simulink model "Ef_c"  (R2017a)
settings: Solver=VariableStepAuto  StartTime=0.0  StopTime=100  RelTol=1e-3
InitFcn:
  | m1 = .35;
  | m2 = 2;
  | l = .5;
  | g = 9.8;
  | ze = l/2;
  | 
  | C1 = 3/(m2*l^2+3*m1*ze^2);
  | 
  | tr_th = 1;
  | h_th = .707;
  | Wn_th = 2.2 / tr_th;
  | kd_th = 2*h_th*Wn_th/C1/l;
  | kp_th = Wn_th^2/(C1*l);
  | 
  | tr_z = 5*tr_th;
  | h = .707;
  | Wn = 2.2 / tr_z;
  | 
  | K = -Wn^2/9.81;
  | a = -K / ((1*h*Wn*1.5+.1)/(1.5*9.81));
  | K = -.022;
  | a = .3;
  | 
  | E_param
undefined symbols (not defined in the file or in its folder): E_animation, P
settings Model: Creator=Mat Haskell  LastModifiedBy=Mat Haskell

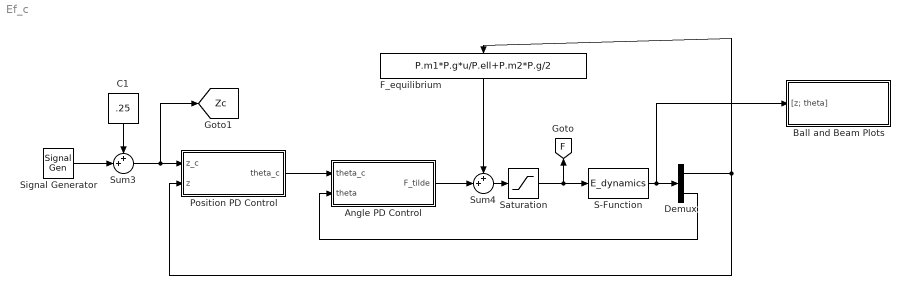
== system Ef_c ==
  Angle PD Control : Subsystem
  Ball and Beam Plots : Subsystem
  C1 : Constant  Value=.25
  Demux : Demux  Outputs=2
  F_equilibrium : Fcn  Expr=P.m1*P.g*u/P.ell+P.m2*P.g/2
  Position PD Control : Subsystem
  S-Function : S-Function  FunctionName=E_dynamics  Parameters=P  SFunctionDeploymentMode=off  EnableBusSupport=off
  Saturation : Saturate  UpperLimit=15  LowerLimit=0
  Signal Generator : SignalGenerator  WaveForm=square  Amplitude=.125  Frequency=.03
  Sum3 : Sum  Inputs=++|
  Sum4 : Sum  Inputs=++|
  tag scope: F=global, Zc=global
  wires:
  Sum4/1 -> Saturation/1
  F_equilibrium/1 -> Sum4/1
  Demux/2 -> Angle PD Control/2(theta)
  Position PD Control/1(theta_c) -> Angle PD Control/1(theta_c)
  Demux/1 -> Position PD Control/2(z), F_equilibrium/1
  Signal Generator/1 -> Sum3/2
  Sum3/1 -> [Zc], Position PD Control/1(z_c)
  Saturation/1 -> S-Function/1, [F]
  Angle PD Control/1(F_tilde) -> Sum4/2
  S-Function/1 -> Demux/1, Ball and Beam Plots/1("[z; theta]")
  C1/1 -> Sum3/1

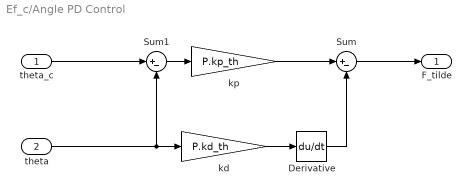
== system Ef_c/Angle PD Control ==
  theta_c : Inport
  theta : Inport  Port=2
  Derivative : Derivative
  Sum : Sum  Inputs=|+-
  Sum1 : Sum  Inputs=|+-
  kd : Gain  Gain=P.kd_th
  kp : Gain  Gain=P.kp_th
  F_tilde : Outport
  wires:
  Derivative/1 -> Sum/2
  Sum1/1 -> kp/1
  theta_c/1 -> Sum1/1
  Sum/1 -> F_tilde/1
  kp/1 -> Sum/1
  kd/1 -> Derivative/1
  theta/1 -> Sum1/2, kd/1

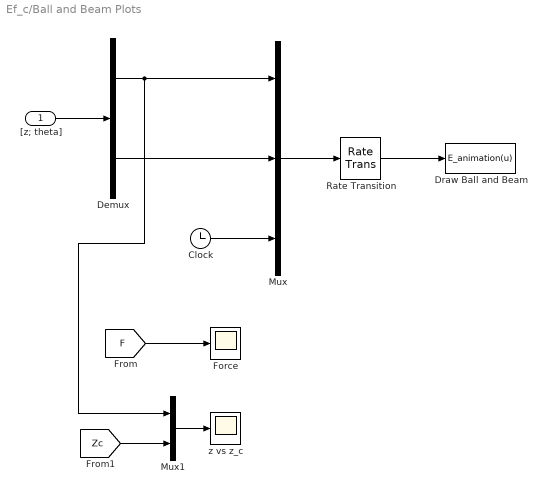
== system Ef_c/Ball and Beam Plots ==
  "[z; theta]" : Inport
  Clock : Clock
  Demux : Demux  Outputs=2
  Draw Ball and Beam : MATLABFcn  MATLABFcn=E_animation(u)  OutputDimensions=0
  Force : Scope
  Mux : Mux  Inputs=3
  Mux1 : Mux  Inputs=2
  Rate Transition : RateTransition  OutPortSampleTime=P.t_plot
  z vs z_c : Scope
  wires:
  "[z; theta]"/1 -> Demux/1
  Rate Transition/1 -> Draw Ball and Beam/1
  Mux/1 -> Rate Transition/1
  Clock/1 -> Mux/3
  Demux/1 -> Mux1/1, Mux/1
  Demux/2 -> Mux/2
  [F] -> Force/1
  Mux1/1 -> z vs z_c/1
  [Zc] -> Mux1/2

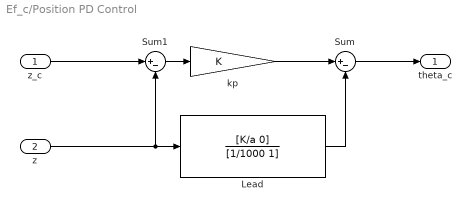
== system Ef_c/Position PD Control ==
  z_c : Inport
  z : Inport  Port=2
  Lead : TransferFcn  Numerator=[K/a 0]  Denominator=[1/1000 1]
  Sum : Sum  Inputs=|+-
  Sum1 : Sum  Inputs=|+-
  kp : Gain  Gain=K
  theta_c : Outport
  wires:
  Sum1/1 -> kp/1
  z_c/1 -> Sum1/1
  Sum/1 -> theta_c/1
  kp/1 -> Sum/1
  z/1 -> Lead/1, Sum1/2
  Lead/1 -> Sum/2
